simulink model "uav_control"  (R2023b)
settings: Solver=ode45  StartTime=0  StopTime=500  RelTol=1e-4
undefined symbols (not defined in the file): Aileron, b, c, C_D, C_l, C_L, C_m, C_n, C_Q, C_T, C_Y, D, Elevator, F_b, i_0, K_Q, K_V, M_b, mass, p, R_motor, Rudder, S, Throttle, V_max
libraries: sharedtransform x2, simulink x2, aerolibsim3d x2, shared6dof x1, sim3dlib x1
settings Model: PauseTimes=10  Creator=Victor  LastModifiedBy=Victor
settings DataIOCC: ExternalInput=getinputstruct(report30)  InitialState=getstatestruct(report30)
settings DebuggingCC: MaxConsecutiveZCsMsg=warning

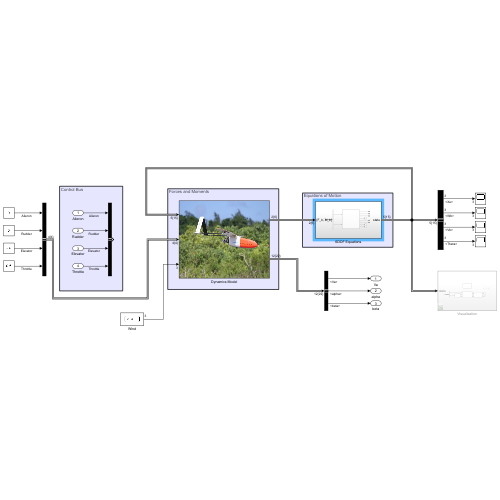
[thumbnail: Simulink's stored preview of the top-level diagram]
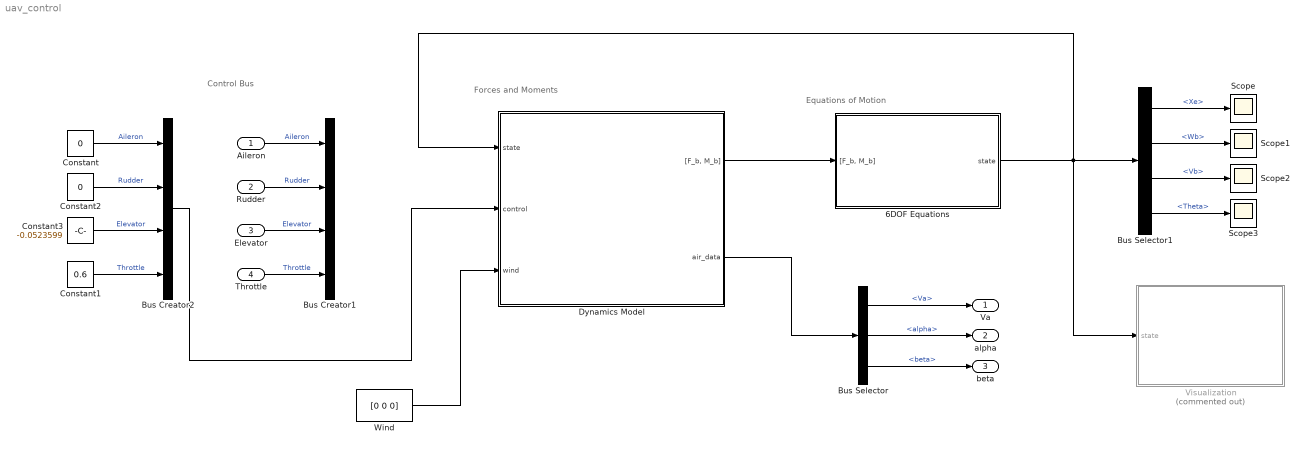
== system uav_control ==
  note: Control Bus
  note: Forces and Moments
  note: Equations of Motion
  Aileron : Inport
  Rudder : Inport  Port=2
  Elevator : Inport  Port=3
  Throttle : Inport  Port=4
  6DOF Equations : Subsystem
  Bus Creator1 : BusCreator  Inputs=Aileron,Rudder,Elevator,Throttle
  Bus Creator2 : BusCreator  Inputs=Aileron,Rudder,Elevator,Throttle
  Bus Selector : BusSelector  OutputSignals=target.Va,target.alpha,target.beta
  Bus Selector1 : BusSelector  OutputSignals=Xe,Wb,Vb,Theta
  Constant : Constant  Value=0
  Constant1 : Constant  Value=0.6
  Constant2 : Constant  Value=0
  Constant3 : Constant  Value=-0.0523599
  Dynamics Model : Subsystem
      mask Display: image('aerosonde_uav.png');
  Scope{,1..3} (4 alike) : Scope
  Visualization : Subsystem  Commented=on
  Wind : Constant  Value=[0 0 0]
  Va : Outport
  alpha : Outport  Port=2
  beta : Outport  Port=3
  wires:
  6DOF Equations/1(state) -> Visualization/1(state), Bus Selector1/1, Dynamics Model/1(state)
  Aileron/1 -> Bus Creator1/1  "Aileron"
  Rudder/1 -> Bus Creator1/2  "Rudder"
  Elevator/1 -> Bus Creator1/3  "Elevator"
  Throttle/1 -> Bus Creator1/4  "Throttle"
  Dynamics Model/1("[F_b, M_b]") -> 6DOF Equations/1("[F_b, M_b]")
  Dynamics Model/2(air_data) -> Bus Selector/1
  Bus Selector/1 -> Va/1  "<Va>"
  Bus Selector1/1 -> Scope/1  "<Xe>"
  Bus Selector1/2 -> Scope1/1  "<Wb>"
  Bus Selector1/3 -> Scope2/1  "<Vb>"
  Bus Selector1/4 -> Scope3/1  "<Theta>"
  Constant1/1 -> Bus Creator2/4  "Throttle"
  Constant/1 -> Bus Creator2/1  "Aileron"
  Constant2/1 -> Bus Creator2/2  "Rudder"
  Constant3/1 -> Bus Creator2/3  "Elevator"
  Bus Creator2/1 -> Dynamics Model/2(control)
  Bus Selector/2 -> alpha/1  "<alpha>"
  Bus Selector/3 -> beta/1  "<beta>"
  Wind/1 -> Dynamics Model/3(wind)

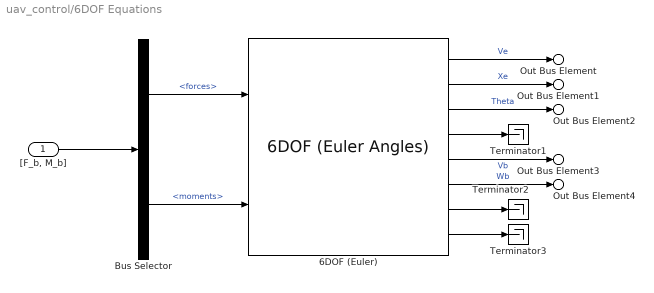
== system uav_control/6DOF Equations ==
  "[F_b, M_b]" : Inport
  6DOF (Euler) : shared6dof/6DOF (Euler Angles)  units=Metric (MKS)  mtype=Fixed  rep=Euler Angles  xme_0=x_0  Vm_0=v_0  eul_0=theta_0  pm_0=w_0  mass_0=mass  mass_e=0.5  mass_f=2.0  inertia=I  inertia_e=eye(3)  inertia_f=2*eye(3)  k_quat=1.0  vre_flag=on  abi_flag=off  aMode=0  xme_statename=''  Vm_statename=''  eul_statename=''  quat_statename=''  pm_statename=''  mass_statename=''
      settings: LibrarySourceBlock=aerolib6dof2/6DOF (Quaternion)
  Bus Selector : BusSelector  OutputSignals=forces,moments
  Terminator1 : Terminator
  Terminator2 : Terminator
  Terminator3 : Terminator
  Out Bus Element : Outport  PortName=state  Element=Ve
  Out Bus Element1 : Outport  PortName=state  Element=Xe
  Out Bus Element2 : Outport  PortName=state  Element=Theta
  Out Bus Element3 : Outport  PortName=state  Element=Vb
  Out Bus Element4 : Outport  PortName=state  Element=Wb
  wires:
  6DOF (Euler)/8 -> Terminator3/1
  6DOF (Euler)/4 -> Terminator1/1
  6DOF (Euler)/7 -> Terminator2/1
  "[F_b, M_b]"/1 -> Bus Selector/1
  Bus Selector/1 -> 6DOF (Euler)/1  "<forces>"
  Bus Selector/2 -> 6DOF (Euler)/2  "<moments>"
  6DOF (Euler)/1 -> Out Bus Element/1  "Ve"
  6DOF (Euler)/2 -> Out Bus Element1/1  "Xe"
  6DOF (Euler)/3 -> Out Bus Element2/1  "Theta"
  6DOF (Euler)/5 -> Out Bus Element3/1  "Vb"
  6DOF (Euler)/6 -> Out Bus Element4/1  "Wb"

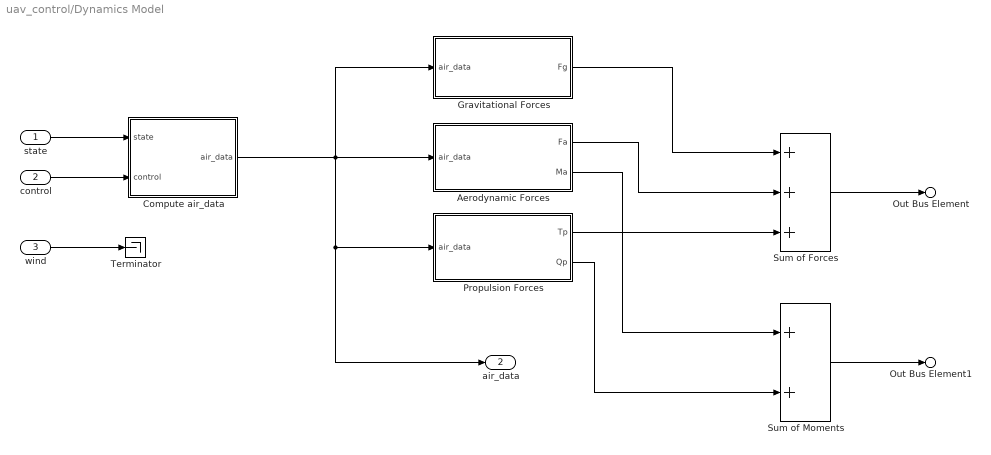
== system uav_control/Dynamics Model ==
  state : Inport
  control : Inport  Port=2
  wind : Inport  Port=3
  Aerodynamic Forces : Subsystem
  Compute air_data : Subsystem
  Gravitational Forces : Subsystem
  Propulsion Forces : Subsystem
  Sum of Forces : Sum  Inputs=+++
  Sum of Moments : Sum
  Terminator : Terminator
  Out Bus Element : Outport  PortName=[F_b, M_b]  Element=forces
  Out Bus Element1 : Outport  PortName=[F_b, M_b]  Element=moments
  air_data : Outport  Port=2
  wires:
  Aerodynamic Forces/2(Ma) -> Sum of Moments/1
  Aerodynamic Forces/1(Fa) -> Sum of Forces/2
  Gravitational Forces/1(Fg) -> Sum of Forces/1
  Sum of Moments/1 -> Out Bus Element1/1
  Sum of Forces/1 -> Out Bus Element/1
  wind/1 -> Terminator/1
  state/1 -> Compute air_data/1(state)
  control/1 -> Compute air_data/2(control)
  Compute air_data/1(air_data) -> Propulsion Forces/1(air_data), air_data/1, Gravitational Forces/1(air_data), Aerodynamic Forces/1(air_data)
  Propulsion Forces/1(Tp) -> Sum of Forces/3
  Propulsion Forces/2(Qp) -> Sum of Moments/2

== system uav_control/Visualization ==
  state : Inport
  Bus Selector : BusSelector  OutputSignals=Xe,Theta
  Compare To Constant : simulink/Logic and Bit Operations/Compare To Constant  Commented=on  relop=<=  const=0  OutDataTypeStr=boolean
  Scope : Scope
  Simulation 3D Aircraft : aerolibsim3d/Simulation 3D Aircraft  Mesh=Sky Hogg  MeshPath=/MathWorksAerospaceContent/Vehicles/Aircraft/Custom/Mesh/SK_HL20.SK_HL20  MeshPathAT=/MathWorksAerospaceContent/Vehicles/Aircraft/AirTransport/Mesh/SK_AirTransport.SK_AirTransport  MeshPathGA=/MathWorksAerospaceContent/Vehicles/Aircraft/GeneralAviation/Mesh/SK_GeneralAviation.SK_GeneralAviation  AircraftColor=Red  ActorName=SimulinkVehicle1  Translation=[0 0 -2000; zeros(10, 3)]  Rotation=zeros(11, 3)  IsGHSensorEnabled=on  AreGHRaysVisible=off  IsOutputReshapeEnabled=off  GHRayLength=2500  GHBodyOffset=0.90  GHFrontTireRadius=0.21  GHLeftTireRadius=0.21  GHRightTireRadius=0.21  WoWSensorTolerance=0.05  LightsConfig=Automatic lights  LandingLightIntensity=300000  LandingLightConeAngle=15  CustomLeftLandingLightLocation=[0 0 0]  CustomLeftLandingLightOrientation=[0 0 0]  CustomRightLandingLightLocation=[0 0 0]  CustomRightLandingLightOrientation=[0 0 0]  TaxiLightIntensity=150000  TaxiLightConeAngle=36  CustomTaxiLightLocation=[0 0 0]  CustomTaxiLightOrientation=[0 0 0]  NavLightIntensity=500  PositionLightIntensity=500  StrobeLightIntensity=5000  WingtipStrobePeriod=1.5  WingtipStrobePulseWidth=6  TailStrobePeriod=1.5  TailStrobePulseWidth=6  BeaconLightIntensity=4000  BeaconPeriod=1.5  BeaconPulseWidth=10  SampleTime=-1  ActorType=SimulinkVehicle  ID=1  aMode=0  ActorTag=SimulinkVehicle1
  Simulation 3D Scene Configuration : sim3dlib/Simulation 3D Scene Configuration  Priority=0  ProjectFormat=Default Scenes  SceneDesc=Airport  ProjectName=C:\Program Files\MATLAB\R2023b\toolbox\shared\sim3d_projects\automotive_project_windows\UE\WindowsNoEditor\VehicleSimulation.exe  ScenePath=/Game/Maps/HwStrght  EnableOpenDRIVE=off  vehTagList={'Custom';'Scene Origin';'SimulinkVehicle1'}  vehTag=SimulinkVehicle1  FreeCameraInitialTranslation=[0, 0, 0]  FreeCameraDefaultInitialTranslation=[-6, 0, 2]  FreeCameraInitialRotation=[0, 0, 0]  FreeCameraDefaultInitialRotation=[0, -15, 0]  OpVisEn=off  Ts=1/60  EnableWindow=on  EnableRemoteAccess=off  EnableWeather=off  SunAltitude=40.0  SunAzimuth=90  clouds=10  wind=1  fog=0  rain=0  EnableGeospatial=off  OriginHeight=200  OriginLatitude=40.744652  OriginLongitude=-73.988864  MapStyle=Aerial  AdditionalAssetIDs=[]  UseAdvancedSunSky=off  SolarTime=11  TimeZone=-5  Day=21  Month=9  Year=2022  UseDaylightSavingTime=on  DSTStartDay=10  DSTStartMonth=3  DSTEndDay=3  DSTEndMonth=11  DSTSwitchHour=2  sensorTag=MainCamera1  sensorId=1  sensorName=MainCamera1  mountLoc=Origin  offsetFlag=off  tmountOffset=[0, 0, 0]  rmountOffset=[0, 0, 0]  HorizontalResolution=1280  VerticalResolution=720  HorizontalFOV=60  mountPoint=[0 0 0]  mountOrientation=[0 0 0]  aMode=0  ID=1  GeoTrigger=Inactive
      settings: LibrarySourceBlock=aerolibsim3d/Simulation 3D Scene Configuration
  Simulation 3D Sky Hogg Pack : aerolibsim3d/Simulation 3D Sky Hogg Pack  Propeller_R=on  Rudder_R=off  Elevator_R=off  Left_Aileron_R=off  Right_Aileron_R=off  Flaps_R=off  Nose_Wheel_Strut_R=off  Nose_Wheel_R=off  Left_Wheel_R=off  Right_Wheel_R=off  AdjustForCesium=off  Heading0=90
  SkyHogg Rotation : Subsystem
  Stop Simulation : Stop  Commented=on
  Terminator : Terminator
  wires:
  Simulation 3D Sky Hogg Pack/1 -> Simulation 3D Aircraft/1
  SkyHogg Rotation/1(Body_R) -> Simulation 3D Sky Hogg Pack/2
  Simulation 3D Sky Hogg Pack/2 -> Simulation 3D Aircraft/2
  Simulation 3D Aircraft/1 -> Scope/1
  SkyHogg Rotation/2(Prop_R) -> Simulation 3D Sky Hogg Pack/3
  Simulation 3D Aircraft/2 -> Terminator/1
  Bus Selector/1 -> Simulation 3D Sky Hogg Pack/1  "<Xe>"
  Bus Selector/2 -> SkyHogg Rotation/1(BodyAngles)  "<Theta>"
  state/1 -> Bus Selector/1
  Compare To Constant/1 -> Stop Simulation/1

== system uav_control/Dynamics Model/Aerodynamic Forces ==
  air_data : Inport
  Add : Sum
  Add1 : Sum
  Lateral Forces : Subsystem
  Longitudinal Forces : Subsystem
  Fa : Outport
  Ma : Outport  Port=2
  wires:
  Add1/1 -> Ma/1
  Longitudinal Forces/2(Ma_b) -> Add1/2
  Lateral Forces/2(MaL_b) -> Add1/1
  Add/1 -> Fa/1
  Longitudinal Forces/1(fa_b) -> Add/2
  Lateral Forces/1(faL_b) -> Add/1
  air_data/1 -> Longitudinal Forces/1(air_data), Lateral Forces/1(air_data)

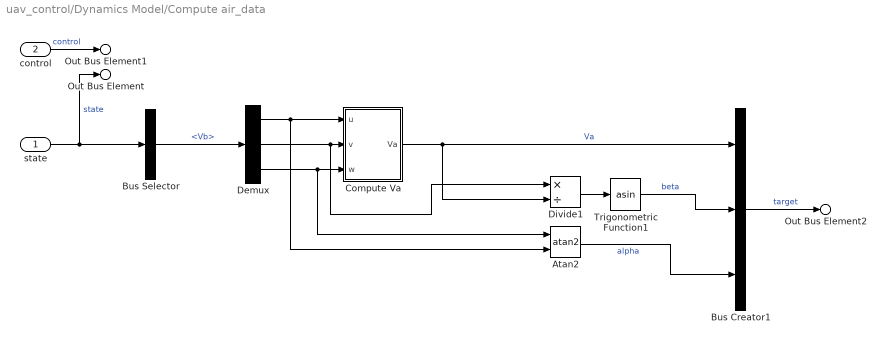
== system uav_control/Dynamics Model/Compute air_data ==
  state : Inport
  control : Inport  Port=2
  Atan2 : Trigonometry  Operator=atan2
  Bus Creator1 : BusCreator  Inputs=3
  Bus Selector : BusSelector  OutputSignals=Vb
  Compute Va : Subsystem
  Demux : Demux  Outputs=3
  Divide1 : Product  Inputs=*/
  Trigonometric Function1 : Trigonometry  Operator=asin
  Out Bus Element : Outport  PortName=air_data  Element=state
  Out Bus Element1 : Outport  PortName=air_data  Element=control
  Out Bus Element2 : Outport  PortName=air_data  Element=target
  wires:
  state/1 -> Out Bus Element/1, Bus Selector/1  "state"
  Trigonometric Function1/1 -> Bus Creator1/2  "beta"
  Divide1/1 -> Trigonometric Function1/1
  Compute Va/1(Va) -> Divide1/2, Bus Creator1/1  "Va"
  Atan2/1 -> Bus Creator1/3  "alpha"
  Demux/2 -> Divide1/1, Compute Va/2(v)
  Demux/1 -> Compute Va/1(u), Atan2/2
  Bus Creator1/1 -> Out Bus Element2/1  "target"
  control/1 -> Out Bus Element1/1  "control"
  Bus Selector/1 -> Demux/1  "<Vb>"
  Demux/3 -> Compute Va/3(w), Atan2/1

== system uav_control/Dynamics Model/Gravitational Forces ==
  air_data : Inport
  Bus Selector : BusSelector  OutputSignals=state.Theta
  Gravity : Gain  Gain=9.81
  Mass : Constant  Value=mass
  NED : Concatenate  NumInputs=3
  Vehicle-frame to Body-frame : Subsystem
  Zero : Constant  Value=0  OutDataTypeStr=Inherit: Inherit via back propagation
  Fg : Outport
  wires:
  Mass/1 -> Gravity/1
  Gravity/1 -> NED/3
  Zero/1 -> NED/1, NED/2
  NED/1 -> Vehicle-frame to Body-frame/2(Fg_v)  "Fg_v"
  Vehicle-frame to Body-frame/1(Fg_b) -> Fg/1
  air_data/1 -> Bus Selector/1
  Bus Selector/1 -> Vehicle-frame to Body-frame/1(Theta)  "<Theta>"

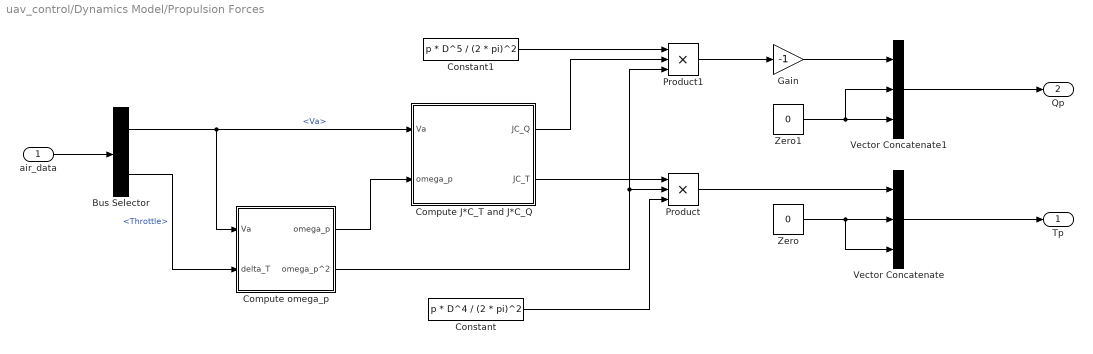
== system uav_control/Dynamics Model/Propulsion Forces ==
  air_data : Inport
  Bus Selector : BusSelector  OutputSignals=target.Va,control.Throttle
  Compute J*C_T and J*C_Q : Subsystem
  Compute omega_p : Subsystem
  Constant : Constant  Value=p * D^4 / (2 * pi)^2
  Constant1 : Constant  Value=p * D^5 / (2 * pi)^2
  Gain : Gain  Gain=-1
  Product : Product  Inputs=3
  Product1 : Product  Inputs=3
  Vector Concatenate : Concatenate  NumInputs=3
  Vector Concatenate1 : Concatenate  NumInputs=3
  Zero : Constant  Value=0  OutDataTypeStr=Inherit: Inherit via back propagation
  Zero1 : Constant  Value=0  OutDataTypeStr=Inherit: Inherit via back propagation
  Tp : Outport
  Qp : Outport  Port=2
  wires:
  Zero/1 -> Vector Concatenate/2, Vector Concatenate/3
  Vector Concatenate/1 -> Tp/1
  Zero1/1 -> Vector Concatenate1/2, Vector Concatenate1/3
  Vector Concatenate1/1 -> Qp/1
  Gain/1 -> Vector Concatenate1/1
  air_data/1 -> Bus Selector/1
  Product/1 -> Vector Concatenate/1
  Product1/1 -> Gain/1
  Compute omega_p/2(omega_p^2) -> Product/2, Product1/3
  Compute omega_p/1(omega_p) -> Compute J*C_T and J*C_Q/2(omega_p)
  Bus Selector/1 -> Compute J*C_T and J*C_Q/1(Va), Compute omega_p/1(Va)  "<Va>"
  Compute J*C_T and J*C_Q/2(JC_T) -> Product/1
  Constant1/1 -> Product1/1
  Bus Selector/2 -> Compute omega_p/2(delta_T)  "<Throttle>"
  Compute J*C_T and J*C_Q/1(JC_Q) -> Product1/2
  Constant/1 -> Product/3

== system uav_control/Visualization/SkyHogg Rotation ==
  BodyAngles : Inport
  Demux : Demux  Outputs=3
  Psi : Constant  Value=0
  Ramp : simulink/Sources/Ramp  slope=157  start=0  InitialOutput=0
  Reshape1 : Reshape  OutputDimensionality=Row vector (2-D)
  Reshape2 : Reshape  OutputDimensionality=Row vector (2-D)
  Theta : Constant  Value=0
  Vector Concatenate : Concatenate  NumInputs=3
  Vector Concatenate3 : Concatenate  NumInputs=3
  Body_R : Outport
  Prop_R : Outport  Port=2
  wires:
  Vector Concatenate/1 -> Reshape1/1  "Body"
  Reshape1/1 -> Body_R/1
  Vector Concatenate3/1 -> Reshape2/1  "Propeller"
  Psi/1 -> Vector Concatenate3/3  "psi"
  Theta/1 -> Vector Concatenate3/2  "theta"
  Ramp/1 -> Vector Concatenate3/1  "phi"
  Reshape2/1 -> Prop_R/1
  BodyAngles/1 -> Demux/1
  Demux/1 -> Vector Concatenate/1
  Demux/2 -> Vector Concatenate/2
  Demux/3 -> Vector Concatenate/3

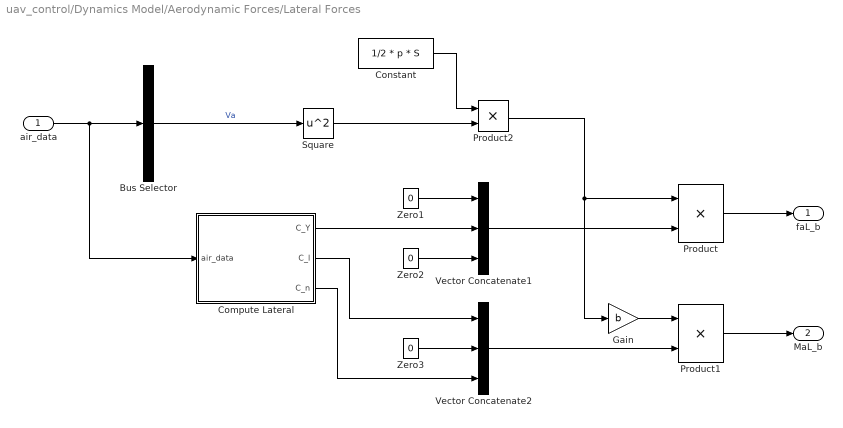
== system uav_control/Dynamics Model/Aerodynamic Forces/Lateral Forces ==
  air_data : Inport
  Bus Selector : BusSelector  OutputSignals=target.Va  OutputAsBus=on
  Compute Lateral : Subsystem
  Constant : Constant  Value=1/2 * p * S
  Gain : Gain  Gain=b
  Product : Product
  Product1 : Product
  Product2 : Product
  Square : Math  Operator=square
  Vector Concatenate1 : Concatenate  NumInputs=3
  Vector Concatenate2 : Concatenate  NumInputs=3
  Zero1 : Constant  Value=0  OutDataTypeStr=Inherit: Inherit via back propagation
  Zero2 : Constant  Value=0  OutDataTypeStr=Inherit: Inherit via back propagation
  Zero3 : Constant  Value=0  OutDataTypeStr=Inherit: Inherit via back propagation
  faL_b : Outport
  MaL_b : Outport  Port=2
  wires:
  Bus Selector/1 -> Square/1  "Va"
  Product/1 -> faL_b/1
  air_data/1 -> Compute Lateral/1(air_data), Bus Selector/1
  Zero1/1 -> Vector Concatenate1/1
  Zero2/1 -> Vector Concatenate1/3
  Compute Lateral/1(C_Y) -> Vector Concatenate1/2
  Compute Lateral/3(C_n) -> Vector Concatenate2/3
  Compute Lateral/2(C_l) -> Vector Concatenate2/1
  Zero3/1 -> Vector Concatenate2/2
  Product1/1 -> MaL_b/1
  Square/1 -> Product2/2
  Constant/1 -> Product2/1
  Product2/1 -> Gain/1, Product/1
  Vector Concatenate1/1 -> Product/2
  Vector Concatenate2/1 -> Product1/2
  Gain/1 -> Product1/1

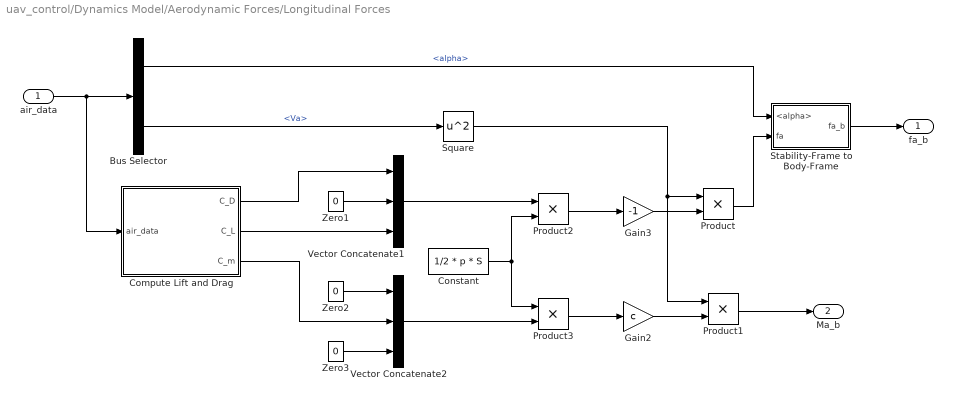
== system uav_control/Dynamics Model/Aerodynamic Forces/Longitudinal Forces ==
  air_data : Inport
  Bus Selector : BusSelector  OutputSignals=target.alpha,target.Va
  Compute Lift and Drag : Subsystem
  Constant : Constant  Value=1/2 * p * S
  Gain2 : Gain  Gain=c
  Gain3 : Gain  Gain=-1
  Product{,1..3} (4 alike) : Product
  Square : Math  Operator=square
  Stability-Frame to Body-Frame : Subsystem
  Vector Concatenate1 : Concatenate  NumInputs=3
  Vector Concatenate2 : Concatenate  NumInputs=3
  Zero1 : Constant  Value=0  OutDataTypeStr=Inherit: Inherit via back propagation
  Zero2 : Constant  Value=0  OutDataTypeStr=Inherit: Inherit via back propagation
  Zero3 : Constant  Value=0  OutDataTypeStr=Inherit: Inherit via back propagation
  fa_b : Outport
  Ma_b : Outport  Port=2
  wires:
  air_data/1 -> Bus Selector/1, Compute Lift and Drag/1(air_data)
  Vector Concatenate1/1 -> Product2/1
  Zero1/1 -> Vector Concatenate1/2
  Compute Lift and Drag/1(C_D) -> Vector Concatenate1/1
  Compute Lift and Drag/2(C_L) -> Vector Concatenate1/3
  Vector Concatenate2/1 -> Product3/2
  Zero3/1 -> Vector Concatenate2/3
  Compute Lift and Drag/3(C_m) -> Vector Concatenate2/2
  Product1/1 -> Ma_b/1
  Bus Selector/2 -> Square/1  "<Va>"
  Bus Selector/1 -> Stability-Frame to Body-Frame/1(<alpha>)  "<alpha>"
  Stability-Frame to Body-Frame/1(fa_b) -> fa_b/1
  Zero2/1 -> Vector Concatenate2/1
  Constant/1 -> Product2/2, Product3/1
  Product2/1 -> Gain3/1
  Product3/1 -> Gain2/1
  Gain2/1 -> Product1/2
  Gain3/1 -> Product/2
  Square/1 -> Product1/1, Product/1
  Product/1 -> Stability-Frame to Body-Frame/2(fa)

== system uav_control/Dynamics Model/Compute air_data/Compute Va ==
  u : Inport
  v : Inport  Port=2
  w : Inport  Port=3
  Add : Sum  Inputs=+++
  Square : Math  Operator=square
  Square Root : Sqrt
  Square1 : Math  Operator=square
  Square2 : Math  Operator=square
  Va : Outport
  wires:
  Square2/1 -> Add/3
  Square/1 -> Add/1
  Add/1 -> Square Root/1
  Square1/1 -> Add/2
  u/1 -> Square/1
  w/1 -> Square2/1
  v/1 -> Square1/1
  Square Root/1 -> Va/1  "Va"

== system uav_control/Dynamics Model/Gravitational Forces/Vehicle-frame to Body-frame ==
  Theta : Inport
  Fg_v : Inport  Port=2
  Matrix Multiply : Product  Multiplication=Matrix(*)
  R^v_b : sharedtransform/Rotation Angles to Direction Cosine Matrix  rotationOrder=ZYX  aMode=aMode
  Reshape : Reshape  OutputDimensionality=Column vector (2-D)
  Reshape1 : Reshape
  Selector : Selector  InputPortWidth=3  IndexOptions=Index vector (dialog)  Indices=[3 2 1]  OutputSizes=1
  Fg_b : Outport
  wires:
  Matrix Multiply/1 -> Reshape1/1
  Theta/1 -> Selector/1
  Selector/1 -> R^v_b/1
  R^v_b/1 -> Matrix Multiply/1
  Fg_v/1 -> Reshape/1
  Reshape/1 -> Matrix Multiply/2
  Reshape1/1 -> Fg_b/1

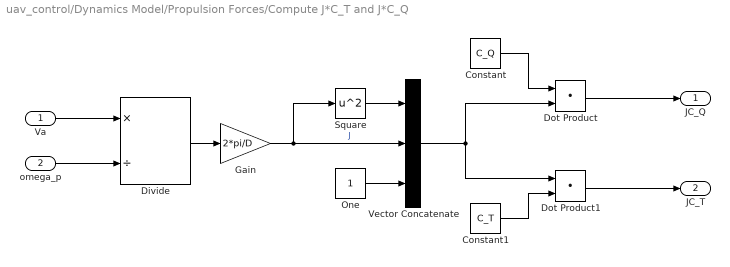
== system uav_control/Dynamics Model/Propulsion Forces/Compute J*C_T and J*C_Q ==
  Va : Inport
  omega_p : Inport  Port=2
  Constant : Constant  Value=C_Q
  Constant1 : Constant  Value=C_T
  Divide : Product  Inputs=*/
  Dot Product : DotProduct  OutDataTypeStr=Inherit: Inherit via internal rule
  Dot Product1 : DotProduct  OutDataTypeStr=Inherit: Inherit via internal rule
  Gain : Gain  Gain=2*pi/D
  One : Constant  OutDataTypeStr=Inherit: Inherit via back propagation
  Square : Math  Operator=square
  Vector Concatenate : Concatenate  NumInputs=3
  JC_Q : Outport
  JC_T : Outport  Port=2
  wires:
  Va/1 -> Divide/1
  omega_p/1 -> Divide/2
  Divide/1 -> Gain/1
  Gain/1 -> Square/1, Vector Concatenate/2  "J"
  Square/1 -> Vector Concatenate/1
  One/1 -> Vector Concatenate/3
  Constant/1 -> Dot Product/1
  Vector Concatenate/1 -> Dot Product1/1, Dot Product/2
  Constant1/1 -> Dot Product1/2
  Dot Product1/1 -> JC_T/1
  Dot Product/1 -> JC_Q/1

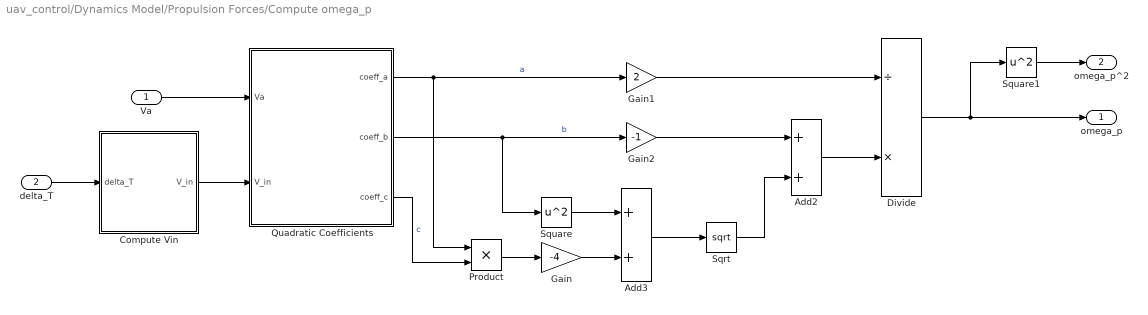
== system uav_control/Dynamics Model/Propulsion Forces/Compute omega_p ==
  Va : Inport
  delta_T : Inport  Port=2
  Add2 : Sum
  Add3 : Sum
  Compute Vin : Subsystem
  Divide : Product  Inputs=/*
  Gain : Gain  Gain=-4
  Gain1 : Gain  Gain=2
  Gain2 : Gain  Gain=-1
  Product : Product
  Quadratic Coefficients : Subsystem
  Sqrt : Sqrt
  Square : Math  Operator=square
  Square1 : Math  Operator=square
  omega_p : Outport
  omega_p^2 : Outport  Port=2
  wires:
  delta_T/1 -> Compute Vin/1(delta_T)
  Product/1 -> Gain/1
  Divide/1 -> omega_p/1, Square1/1
  Va/1 -> Quadratic Coefficients/1(Va)
  Compute Vin/1(V_in) -> Quadratic Coefficients/2(V_in)
  Square1/1 -> omega_p^2/1
  Quadratic Coefficients/1(coeff_a) -> Product/1, Gain1/1  "a"
  Gain1/1 -> Divide/1
  Quadratic Coefficients/2(coeff_b) -> Square/1, Gain2/1  "b"
  Gain2/1 -> Add2/1
  Sqrt/1 -> Add2/2
  Add3/1 -> Sqrt/1
  Square/1 -> Add3/1
  Gain/1 -> Add3/2
  Quadratic Coefficients/3(coeff_c) -> Product/2  "c"
  Add2/1 -> Divide/2

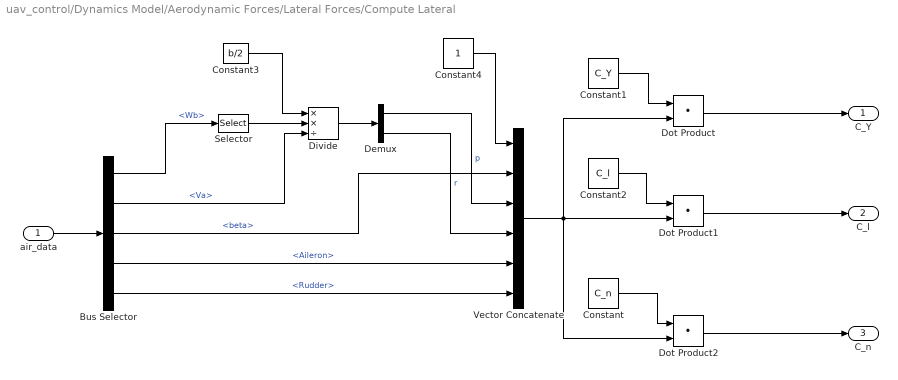
== system uav_control/Dynamics Model/Aerodynamic Forces/Lateral Forces/Compute Lateral ==
  air_data : Inport
  Bus Selector : BusSelector  OutputSignals=state.Wb,target.Va,target.beta,control.Aileron,control.Rudder
  Constant : Constant  Value=C_n
  Constant1 : Constant  Value=C_Y
  Constant2 : Constant  Value=C_l
  Constant3 : Constant  Value=b/2
  Constant4 : Constant
  Demux : Demux  Outputs=2
  Divide : Product  Inputs=**/
  Dot Product : DotProduct  OutDataTypeStr=Inherit: Inherit via internal rule
  Dot Product1 : DotProduct  OutDataTypeStr=Inherit: Inherit via internal rule
  Dot Product2 : DotProduct  OutDataTypeStr=Inherit: Inherit via internal rule
  Selector : Selector  InputPortWidth=3  IndexOptions=Index vector (dialog)  Indices=[1 3]  OutputSizes=1
  Vector Concatenate : Concatenate  NumInputs=6
  C_Y : Outport
  C_l : Outport  Port=2
  C_n : Outport  Port=3
  wires:
  air_data/1 -> Bus Selector/1
  Constant1/1 -> Dot Product/1
  Vector Concatenate/1 -> Dot Product2/2, Dot Product1/2, Dot Product/2
  Constant2/1 -> Dot Product1/1
  Dot Product/1 -> C_Y/1
  Dot Product1/1 -> C_l/1
  Dot Product2/1 -> C_n/1
  Selector/1 -> Divide/2
  Constant4/1 -> Vector Concatenate/1
  Demux/1 -> Vector Concatenate/3  "p"
  Demux/2 -> Vector Concatenate/4  "r"
  Divide/1 -> Demux/1
  Constant/1 -> Dot Product2/1
  Bus Selector/1 -> Selector/1  "<Wb>"
  Bus Selector/2 -> Divide/3  "<Va>"
  Bus Selector/3 -> Vector Concatenate/2  "<beta>"
  Bus Selector/4 -> Vector Concatenate/5  "<Aileron>"
  Bus Selector/5 -> Vector Concatenate/6  "<Rudder>"
  Constant3/1 -> Divide/1

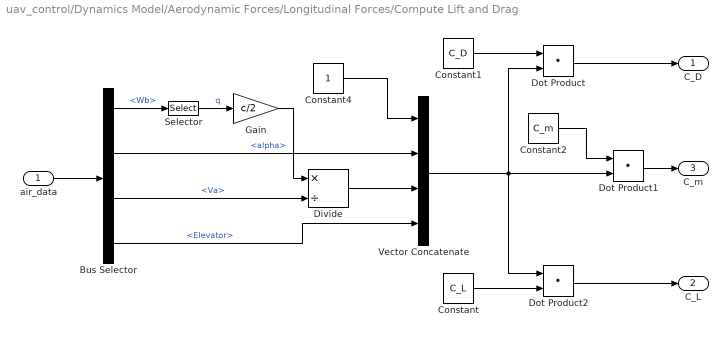
== system uav_control/Dynamics Model/Aerodynamic Forces/Longitudinal Forces/Compute Lift and Drag ==
  air_data : Inport
  Bus Selector : BusSelector  OutputSignals=state.Wb,target.alpha,target.Va,control.Elevator
  Constant : Constant  Value=C_L
  Constant1 : Constant  Value=C_D
  Constant2 : Constant  Value=C_m
  Constant4 : Constant
  Divide : Product  Inputs=*/
  Dot Product : DotProduct  OutDataTypeStr=Inherit: Inherit via internal rule
  Dot Product1 : DotProduct  OutDataTypeStr=Inherit: Inherit via internal rule
  Dot Product2 : DotProduct  OutDataTypeStr=Inherit: Inherit via internal rule
  Gain : Gain  Gain=c/2
  Selector : Selector  InputPortWidth=3  IndexOptions=Index vector (dialog)  Indices=[2]  OutputSizes=1
  Vector Concatenate : Concatenate  NumInputs=4
  C_D : Outport
  C_L : Outport  Port=2
  C_m : Outport  Port=3
  wires:
  Constant4/1 -> Vector Concatenate/1
  air_data/1 -> Bus Selector/1
  Bus Selector/2 -> Vector Concatenate/2  "<alpha>"
  Bus Selector/3 -> Divide/2  "<Va>"
  Gain/1 -> Divide/1
  Divide/1 -> Vector Concatenate/3
  Bus Selector/4 -> Vector Concatenate/4  "<Elevator>"
  Constant1/1 -> Dot Product/1
  Vector Concatenate/1 -> Dot Product2/1, Dot Product1/2, Dot Product/2
  Constant/1 -> Dot Product2/2
  Constant2/1 -> Dot Product1/1
  Dot Product/1 -> C_D/1
  Dot Product1/1 -> C_m/1
  Dot Product2/1 -> C_L/1
  Selector/1 -> Gain/1  "q"
  Bus Selector/1 -> Selector/1  "<Wb>"

== system uav_control/Dynamics Model/Aerodynamic Forces/Longitudinal Forces/Stability-Frame to Body-Frame ==
  <alpha> : Inport
  fa : Inport  Port=2
  Rotation Angles to Direction Cosine Matrix : sharedtransform/Rotation Angles to Direction Cosine Matrix  rotationOrder=ZYX  aMode=aMode
  Stability-Frame to Body-Frame : Product  Multiplication=Matrix(*)
  Vector Concatenate : Concatenate  NumInputs=3
  Zero : Constant  Value=0  OutDataTypeStr=Inherit: Inherit via back propagation
  fa_b : Outport
  wires:
  <alpha>/1 -> Vector Concatenate/2
  Rotation Angles to Direction Cosine Matrix/1 -> Stability-Frame to Body-Frame/1  "R^s_b"
  Zero/1 -> Vector Concatenate/3, Vector Concatenate/1
  Vector Concatenate/1 -> Rotation Angles to Direction Cosine Matrix/1  "[0, a, 0]"
  fa/1 -> Stability-Frame to Body-Frame/2
  Stability-Frame to Body-Frame/1 -> fa_b/1

== system uav_control/Dynamics Model/Propulsion Forces/Compute omega_p/Compute Vin ==
  delta_T : Inport
  Product : Product
  V_max : Constant  Value=V_max
  V_in : Outport
  wires:
  V_max/1 -> Product/2
  Product/1 -> V_in/1
  delta_T/1 -> Product/1

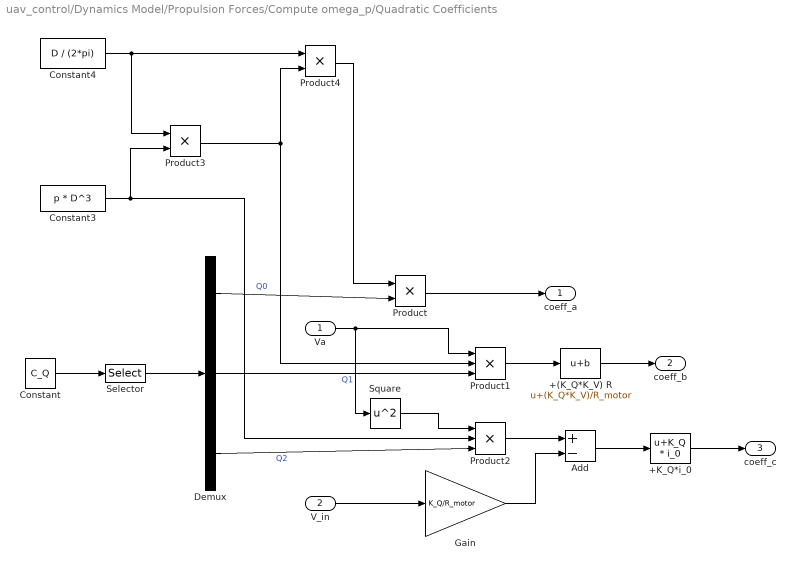
== system uav_control/Dynamics Model/Propulsion Forces/Compute omega_p/Quadratic Coefficients ==
  Va : Inport
  V_in : Inport  Port=2
  +(K_Q*K_V) R : Bias  Bias=(K_Q*K_V)/R_motor  SaturateOnIntegerOverflow=off
  +K_Q*i_0 : Bias  Bias=K_Q * i_0  SaturateOnIntegerOverflow=off
  Add : Sum  Inputs=+-
  Constant : Constant  Value=C_Q
  Constant3 : Constant  Value=p * D^3
  Constant4 : Constant  Value=D / (2*pi)
  Demux : Demux  Outputs=3
  Gain : Gain  Gain=K_Q/R_motor
  Product : Product
  Product1 : Product  Inputs=3
  Product2 : Product  Inputs=3
  Product3 : Product
  Product4 : Product
  Selector : Selector  InputPortWidth=3  IndexOptions=Index vector (dialog)  Indices=[3 2 1]  OutputSizes=1
  Square : Math  Operator=square
  coeff_a : Outport
  coeff_b : Outport  Port=2
  coeff_c : Outport  Port=3
  wires:
  Constant3/1 -> Product2/2, Product3/2
  Constant4/1 -> Product4/1, Product3/1
  Product3/1 -> Product1/2, Product4/2
  Constant/1 -> Selector/1
  Selector/1 -> Demux/1
  Demux/1 -> Product/2  "Q0"
  Demux/2 -> Product1/3  "Q1"
  Demux/3 -> Product2/3  "Q2"
  Product4/1 -> Product/1
  Product/1 -> coeff_a/1
  Va/1 -> Square/1, Product1/1
  Product1/1 -> +(K_Q*K_V) R/1
  +(K_Q*K_V) R/1 -> coeff_b/1
  Square/1 -> Product2/1
  Product2/1 -> Add/1
  V_in/1 -> Gain/1
  Gain/1 -> Add/2
  Add/1 -> +K_Q*i_0/1
  +K_Q*i_0/1 -> coeff_c/1
